simulink subsystem "InvertedPendulum"  (R2024a)
settings: Solver=VariableStepAuto  StartTime=0.0  StopTime=10.0  RelTol=1e-3
undefined symbols (not defined in the file): g, l
settings Model: Creator=nacer  LastModifiedBy=nacer

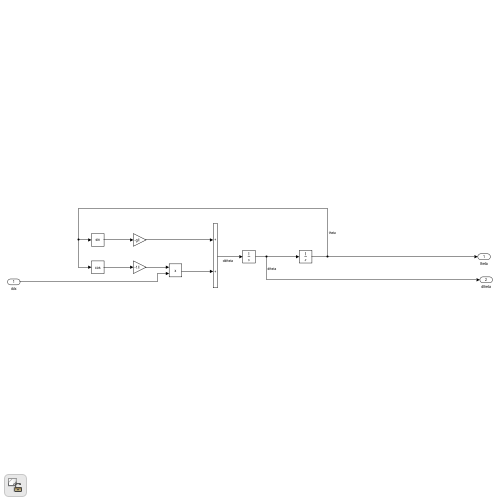
[thumbnail: Simulink's stored preview of the top-level diagram]
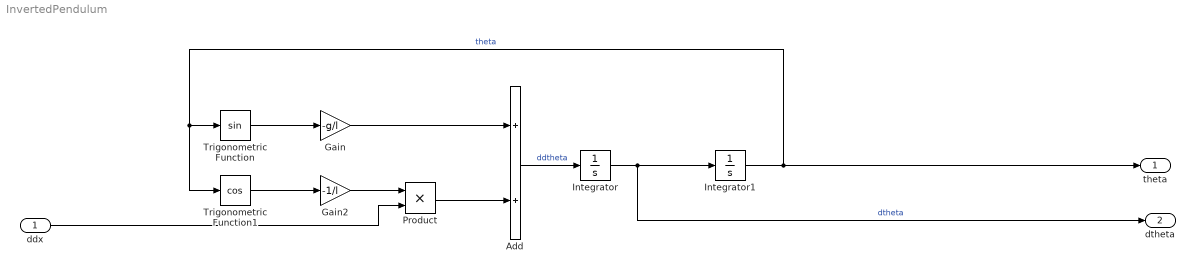
== system InvertedPendulum ==
  ddx : Inport
  Add : Sum
  Gain : Gain  Gain=-g/l
  Gain2 : Gain  Gain=-1/l
  Integrator : Integrator
  Integrator1 : Integrator  InitialCondition=pi*0.9
  Product : Product
  Trigonometric Function : Trigonometry
  Trigonometric Function1 : Trigonometry  Operator=cos
  theta : Outport
  dtheta : Outport  Port=2
  wires:
  Add/1 -> Integrator/1  "ddtheta"
  Integrator1/1 -> Trigonometric Function1/1, Trigonometric Function/1, theta/1  "theta"
  Gain/1 -> Add/1
  Integrator/1 -> Integrator1/1, dtheta/1  "dtheta"
  Product/1 -> Add/2
  Trigonometric Function1/1 -> Gain2/1
  ddx/1 -> Product/2
  Gain2/1 -> Product/1
  Trigonometric Function/1 -> Gain/1
